simulink model "Motor_ctrl"  (R2025b)
settings: Solver=ode15s  StopTime=Tend_sim  FixedStep=Ts/10  MaxStep=Tstep  AbsTol=1e-3  EnableMultiTasking=on
InitFcn:
  | if ~exist('flagwp')
  |     tic
  |     init_sim
  | end
  | mex Motor_ctrl.c User_functions/Src/*.c
StopFcn:
  | % if ~exist('flagwp')
  |   elapsed_time=toc
  | % end
  | %plot_out_sim
values from neighbouring files (symbols this model uses):
  accel = 30000    [init_sim.m]
  Bm = 0.02    [init_sim.m]
  Clarke_inv = [1 0;-0.5 sqrt(3)/2;-0.5 -sqrt(3)/2]    [init_sim.m]
  Ctrl_strategy = 1    [init_sim.m]
  Ctrl_type = 3    [init_sim.m]
  dem = 1    [init_sim.m]
  dT = motorModel.SyreDrive.Converter.dT * 1e-6    [init_sim.m]
  EV_mode = 0    [init_sim.m]
  expC = motorModel.IronPMLossMap_dq.expC    [init_sim.m]
  expH = motorModel.IronPMLossMap_dq.expH    [init_sim.m]
  expPM = motorModel.IronPMLossMap_dq.expPM    [init_sim.m]
  Fd0 = interp2(motorModel.FluxMap_dq.Id,motorModel.FluxMap_dq.Iq,motorModel.FluxMap_dq.Fd,0,0)    [init_sim.m]
  fD_pu_norm = motorModel.FluxMapInv_dq.fD_pu_norm    [init_sim.m]
  fD_vct_max = motorModel.FluxMapInv_dq.fD_vct_max    [init_sim.m]
  fD_vct_ref = motorModel.FluxMapInv_dq.fD_vct_ref    [init_sim.m]
  Fm = interp2(Idd,Iqq,Fdd,0,0)    [init_sim.m]
  fQ_pu_norm = motorModel.FluxMapInv_dq.fQ_pu_norm    [init_sim.m]
  fQ_vct_max = motorModel.FluxMapInv_dq.fQ_vct_max    [init_sim.m]
  fQ_vct_ref = motorModel.FluxMapInv_dq.fQ_vct_ref    [init_sim.m]
  HS_ctrl = 1    [init_sim.m]
  Id_dqt = interpn(motorModel.FluxMapInv_dqt.dataF.Fd,motorModel.FluxMapInv_dqt.dataF.Fq,motorModel.FluxMapInv_dqt.dataF.th,motorModel.FluxMapInv_dqt.dataF.Id,Fd_dqt,Fq_dqt,th_dqt,'cubic')    [init_sim.m]
  Id_fe = motorModel.IronPMLossMap_dq.Id    [init_sim.m]
  iD_pu_norm = motorModel.FluxMapInv_dq.iD_pu_norm    [init_sim.m]
  idRef = interp1(abs(MTPA.id+1i*MTPA.iq),MTPA.id,i0)    [init_sim.m]
  InitIntg_d = Fm*cos(th0)    [init_sim.m]
  InitIntg_q = Fm*sin(th0)    [init_sim.m]
  inj_waveform = 1    [init_sim.m]
  Iq_dqt = interpn(motorModel.FluxMapInv_dqt.dataF.Fd,motorModel.FluxMapInv_dqt.dataF.Fq,motorModel.FluxMapInv_dqt.dataF.th,motorModel.FluxMapInv_dqt.dataF.Iq,Fd_dqt,Fq_dqt,th_dqt,'cubic')    [init_sim.m]
  Iq_fe = motorModel.IronPMLossMap_dq.Iq    [init_sim.m]
  iQ_pu_norm = motorModel.FluxMapInv_dq.iQ_pu_norm    [init_sim.m]
  iqRef = interp1(abs(MTPA.id+1i*MTPA.iq),MTPA.iq,i0)    [init_sim.m]
  IronLoss = 1    [init_sim.m]
  J = 2.7    [init_sim.m]
  motorModelType = motorModel.SyreDrive.modelSetup.motorModelType    [init_sim.m]
  n0 = motorModel.IronPMLossMap_dq.n0    [init_sim.m]
  nRef = 1000    [init_sim.m]
  p = motorModel.data.p    [init_sim.m]
  Pfe_c = motorModel.IronPMLossMap_dq.Pfes_c + motorModel.IronPMLossMap_dq.Pfer_c    [init_sim.m]
  Pfe_h = motorModel.IronPMLossMap_dq.Pfes_h + motorModel.IronPMLossMap_dq.Pfer_h    [init_sim.m]
  Ppm = motorModel.IronPMLossMap_dq.Ppm    [init_sim.m]
  Quad_Maps = 2    [init_sim.m]
  Rs = motorModel.data.Rs    [init_sim.m]
  SS_on = 1    [init_sim.m]
  T0 = interp2(motorModel.FluxMap_dq.Id,motorModel.FluxMap_dq.Iq,motorModel.FluxMap_dq.T,idRef,iqRef)    [init_sim.m]
  T_dqt = interpn(motorModel.FluxMapInv_dqt.dataF.Fd,motorModel.FluxMapInv_dqt.dataF.Fq,motorModel.FluxMapInv_dqt.dataF.th,motorModel.FluxMapInv_dqt.dataF.T,Fd_dqt,Fq_dqt,th_dqt,'cubic')    [init_sim.m]
  Tf = 6    [init_sim.m]
  th0 = 0    [init_sim.m]
  th_max = max(motorModel.FluxMapInv_dqt.dataF.th,[],'all')    [init_sim.m]
  th_min = min(motorModel.FluxMapInv_dqt.dataF.th,[],'all')    [init_sim.m]
  Ts = 1/motorModel.SyreDrive.Converter.fPWM    [init_sim.m]
  Tv = 7.1e-6    (= 7.1e-06)    [init_sim.m]
  VDC = motorModel.data.Vdc    [init_sim.m]
undefined symbols (not defined in the file or in its folder): ACloss, eMotor, interpn, J_rot, magnitude, n0_inv
libraries: nesl_utility x31, fl_lib x26, simulink x10, ee_lib x8, eeTransforms x1
(part 3 of 4)

== system Motor_ctrl/Power block - Inverter + Motor/Noncircuital/FM/Motor Model/Inverse Flux Maps/2D LUT/dq Model/SyR ==
  Vabc : Inport
  theta_elt : Inport  Port=2
  we : Inport  Port=3
  Add : Sum  Inputs=-+-
  Constant : Constant  Value=0
  Demux1 : Demux  Outputs=3
  "Fdq -> idq" : Subsystem
  Gain1 : Gain  Gain=J_rot  Multiplication=Matrix(K*u)
  Gain3 : Gain  Gain=1/p
  Integrator : Integrator  InitialCondition=[Fd0 0]
  Mux1 : Mux  Inputs=2
  Product : Product
  Product2 : Product
  Subsystem1 : Subsystem
  Terminator : Terminator
  ab->dq1 : Subsystem
      mask Display: disp('A(-theta)')
  abc->ab0 : Subsystem
  idq : Outport
  T : Outport  Port=2
  i0 : Outport  Port=3
  Fdq : Outport  Port=4
  wires:
  Subsystem1/1(SinCos) -> ab->dq1/2(sin,cos)
  Product/1 -> Add/3
  theta_elt/1 -> Gain3/1
  Mux1/1 -> ab->dq1/1(X_ab)
  Integrator/1 -> "Fdq -> idq"/1(Fdq), Fdq/1, Gain1/1
  Gain1/1 -> Product/1
  Vabc/1 -> abc->ab0/1(eabc)
  Gain3/1 -> Subsystem1/1(theta_r)
  ab->dq1/1(X_dq) -> Add/2
  abc->ab0/1(eab0) -> Demux1/1
  "Fdq -> idq"/1(idq) -> Product2/2, idq/1
  Demux1/1 -> Mux1/1
  Add/1 -> Integrator/1
  [Rs] -> Product2/1
  Demux1/2 -> Mux1/2
  "Fdq -> idq"/2(T) -> T/1
  Product2/1 -> Add/1
  we/1 -> Product/2
  Constant/1 -> i0/1
  Demux1/3 -> Terminator/1

== system Motor_ctrl/Power block - Inverter + Motor/Noncircuital/FM/Motor Model/Inverse Flux Maps/3D LUTs/Variant Subsystem/IPM ==
  Vabc : Inport
  theta_elt : Inport  Port=2
  we : Inport  Port=3
  Add : Sum  Inputs=-+-
  Constant : Constant  Value=0
  Demux1 : Demux  Outputs=3
  "Fdq -> idq" : Subsystem
      settings: PortSchema="{\"entries\":[{\"content\":{\"sides\":[{\"content\":{\"connectorIds\":[\"In1\"]},\"type\":\"ConnectorPlacement.EquallySpacedRectSide\",\"uuid\":\"c4c89702-6ed2-4f3f-ac47-63a7def21c28\"},{\"content\":{\"connectorIds\":[\"Out1\",\"Out2\"],\"side\":\"RIGHT\"},\"type\":\"ConnectorPlacement.EquallySpacedRectSide\",\"uuid\":\"78e6e96f-e01c-41b0-b9cc-2e557d2d3e77\"},{\"content\":{\"side\":\"TOP\"},\"type\":\"ConnectorPlacement.EquallySpacedRectSide\",\"uuid\":\"5ba1a012-9577-477d-841c-cd762f3f0080\"},{\"content\":{\"connectorIds\":[\"In2\"],\"side\":\"BOTTOM\"},\"type\":\"ConnectorPlacement.EquallySpacedRectSide\",\"uuid\":\"5a42fb6c-9e1a-4def-8312-83961c7d32ea\"}]},\"type\":\"ConnectorPlacement.EquallySpacedConnector\",\"uuid\":\"db03f8b0-b4f5-4aab-82fc-8dea803a4789\"}],\"packageUris\":[\"http://schema.mathworks.com/mf0/Connector/R2020b\"],\"version\":\"1.0\"}"
  Gain1 : Gain  Gain=J_rot  Multiplication=Matrix(K*u)
  Gain3 : Gain  Gain=1/p
  Integrator : Integrator  InitialCondition=[Fd0 0]
  Mux1 : Mux  Inputs=2
  Product : Product
  Product1 : Product
  Subsystem1 : Subsystem
  Terminator : Terminator
  ab->dq1 : Subsystem
      mask Display: disp('A(-theta)')
  abc->ab0 : Subsystem
  idq : Outport
  T : Outport  Port=2
  i0 : Outport  Port=3
  Fdq : Outport  Port=4
  wires:
  theta_elt/1 -> "Fdq -> idq"/2(th_e), Gain3/1
  Product1/1 -> Add/1
  Gain1/1 -> Product/1
  we/1 -> Product/2
  Product/1 -> Add/3
  Add/1 -> Integrator/1
  Integrator/1 -> Fdq/1, "Fdq -> idq"/1(Fdq), Gain1/1
  "Fdq -> idq"/1(idq) -> Product1/2, idq/1
  "Fdq -> idq"/2(T) -> T/1
  [Rs] -> Product1/1
  Vabc/1 -> abc->ab0/1(eabc)
  Gain3/1 -> Subsystem1/1(theta_r)
  abc->ab0/1(eab0) -> Demux1/1
  Subsystem1/1(SinCos) -> ab->dq1/2(sin,cos)
  Demux1/2 -> Mux1/2
  Mux1/1 -> ab->dq1/1(X_ab)
  Demux1/1 -> Mux1/1
  ab->dq1/1(X_dq) -> Add/2
  Constant/1 -> i0/1
  Demux1/3 -> Terminator/1

== system Motor_ctrl/Power block - Inverter + Motor/Noncircuital/FM/Motor Model/Inverse Flux Maps/3D LUTs/Variant Subsystem/PM-SyR ==
  Vabc : Inport
  theta_elt : Inport  Port=2
  we : Inport  Port=3
  Add : Sum  Inputs=-+-
  Constant : Constant  Value=0
  Demux1 : Demux  Outputs=3
  "Fdq -> idq" : Subsystem
      settings: PortSchema="{\"entries\":[{\"content\":{\"sides\":[{\"content\":{\"connectorIds\":[\"In1\"]},\"type\":\"ConnectorPlacement.EquallySpacedRectSide\",\"uuid\":\"658e0025-c3b4-4188-99f2-cbeabc2b5232\"},{\"content\":{\"connectorIds\":[\"Out1\",\"Out2\"],\"side\":\"RIGHT\"},\"type\":\"ConnectorPlacement.EquallySpacedRectSide\",\"uuid\":\"553a685c-efe6-4f4b-af8f-d6d55fb3aed3\"},{\"content\":{\"side\":\"TOP\"},\"type\":\"ConnectorPlacement.EquallySpacedRectSide\",\"uuid\":\"e1cc6d12-3f22-4810-870a-14518fddf4c6\"},{\"content\":{\"connectorIds\":[\"In2\"],\"side\":\"BOTTOM\"},\"type\":\"ConnectorPlacement.EquallySpacedRectSide\",\"uuid\":\"8fa353db-c23e-4667-be44-c63eaefe25e8\"}]},\"type\":\"ConnectorPlacement.EquallySpacedConnector\",\"uuid\":\"5d87f386-f61d-410e-9580-edc792fe8ce3\"}],\"packageUris\":[\"http://schema.mathworks.com/mf0/Connector/R2020b\"],\"version\":\"1.0\"}"
  Gain1 : Gain  Gain=J_rot  Multiplication=Matrix(K*u)
  Gain3 : Gain  Gain=1/p
  Integrator : Integrator  InitialCondition=[Fd0 0]
  Mux1 : Mux  Inputs=2
  Product : Product
  Product1 : Product
  Subsystem1 : Subsystem
  Terminator : Terminator
  ab->dq1 : Subsystem
      mask Display: disp('A(-theta)')
  abc->ab0 : Subsystem
  idq : Outport
  T : Outport  Port=2
  i0 : Outport  Port=3
  Fdq : Outport  Port=4
  wires:
  we/1 -> Product/2
  Subsystem1/1(SinCos) -> ab->dq1/2(sin,cos)
  Mux1/1 -> ab->dq1/1(X_ab)
  Gain1/1 -> Product/1
  Product/1 -> Add/3
  abc->ab0/1(eab0) -> Demux1/1
  ab->dq1/1(X_dq) -> Add/2
  [Rs] -> Product1/1
  "Fdq -> idq"/2(T) -> T/1
  Demux1/1 -> Mux1/1
  Product1/1 -> Add/1
  Demux1/3 -> Terminator/1
  Gain3/1 -> Subsystem1/1(theta_r)
  Integrator/1 -> "Fdq -> idq"/1(Fdq), Fdq/1, Gain1/1
  "Fdq -> idq"/1(idq) -> Product1/2, idq/1
  Demux1/2 -> Mux1/2
  Add/1 -> Integrator/1
  Vabc/1 -> abc->ab0/1(eabc)
  theta_elt/1 -> Gain3/1, "Fdq -> idq"/2(theta_elt)
  Constant/1 -> i0/1

== system Motor_ctrl/Power block - Inverter + Motor/Noncircuital/FM/Motor Model/Inverse Flux Maps/3D LUTs/Variant Subsystem/SyR ==
  Vabc : Inport
  theta_elt : Inport  Port=2
  we : Inport  Port=3
  Add : Sum  Inputs=-+-
  Constant : Constant  Value=0
  Demux1 : Demux  Outputs=3
  "Fdq -> idq" : Subsystem
      settings: PortSchema="{\"entries\":[{\"content\":{\"sides\":[{\"content\":{\"connectorIds\":[\"In1\"]},\"type\":\"ConnectorPlacement.EquallySpacedRectSide\",\"uuid\":\"658e0025-c3b4-4188-99f2-cbeabc2b5232\"},{\"content\":{\"connectorIds\":[\"Out1\",\"Out2\"],\"side\":\"RIGHT\"},\"type\":\"ConnectorPlacement.EquallySpacedRectSide\",\"uuid\":\"553a685c-efe6-4f4b-af8f-d6d55fb3aed3\"},{\"content\":{\"side\":\"TOP\"},\"type\":\"ConnectorPlacement.EquallySpacedRectSide\",\"uuid\":\"e1cc6d12-3f22-4810-870a-14518fddf4c6\"},{\"content\":{\"connectorIds\":[\"In2\"],\"side\":\"BOTTOM\"},\"type\":\"ConnectorPlacement.EquallySpacedRectSide\",\"uuid\":\"ed75ffcc-b3fe-4912-8b15-453be7565ae7\"}]},\"type\":\"ConnectorPlacement.EquallySpacedConnector\",\"uuid\":\"5d87f386-f61d-410e-9580-edc792fe8ce3\"}],\"packageUris\":[\"http://schema.mathworks.com/mf0/Connector/R2020b\"],\"version\":\"1.0\"}"
  Gain1 : Gain  Gain=J_rot  Multiplication=Matrix(K*u)
  Gain3 : Gain  Gain=1/p
  Integrator : Integrator  InitialCondition=[Fd0 0]
  Mux1 : Mux  Inputs=2
  Product : Product
  Product1 : Product
  Subsystem1 : Subsystem
  Terminator : Terminator
  ab->dq1 : Subsystem
      mask Display: disp('A(-theta)')
  abc->ab0 : Subsystem
  idq : Outport
  T : Outport  Port=2
  i0 : Outport  Port=3
  Fdq : Outport  Port=4
  wires:
  we/1 -> Product/2
  Subsystem1/1(SinCos) -> ab->dq1/2(sin,cos)
  Mux1/1 -> ab->dq1/1(X_ab)
  Gain1/1 -> Product/1
  Product/1 -> Add/3
  abc->ab0/1(eab0) -> Demux1/1
  ab->dq1/1(X_dq) -> Add/2
  [Rs] -> Product1/1
  "Fdq -> idq"/2(T) -> T/1
  Demux1/1 -> Mux1/1
  Product1/1 -> Add/1
  Gain3/1 -> Subsystem1/1(theta_r)
  Integrator/1 -> "Fdq -> idq"/1(Fdq), Fdq/1, Gain1/1
  "Fdq -> idq"/1(idq) -> Product1/2, idq/1
  Demux1/2 -> Mux1/2
  Add/1 -> Integrator/1
  Vabc/1 -> abc->ab0/1(eabc)
  theta_elt/1 -> "Fdq -> idq"/2(theta_elt), Gain3/1
  Constant/1 -> i0/1
  Demux1/3 -> Terminator/1

== system Motor_ctrl/Power block - Inverter + Motor/Noncircuital/FM/Motor Model/Iron Losses Maps/Iron Losses/Iron loss Maps/Speed Adaptation ==
  n_m : Inport
  Constant : Constant  Value=n0
  Constant1 : Constant  Value=expC
  Constant2 : Constant  Value=expH
  Constant3 : Constant  Value=expPM
  Divide : Product  Inputs=*/
  Math Function : Math  Operator=pow  SignedPower=on
  Math Function1 : Math  Operator=pow  SignedPower=on
  Math Function2 : Math  Operator=pow  SignedPower=on
  H : Outport
  C : Outport  Port=2
  PM : Outport  Port=3
  wires:
  Math Function2/1 -> PM/1
  Math Function/1 -> H/1
  Constant1/1 -> Math Function1/2
  Divide/1 -> Math Function/1, Math Function1/1, Math Function2/1
  Math Function1/1 -> C/1
  Constant/1 -> Divide/2
  Constant2/1 -> Math Function/2
  Constant3/1 -> Math Function2/2
  n_m/1 -> Divide/1

== system Motor_ctrl/Power block - Inverter + Motor/Circuital/Motor model/CCG model/Motor Model/Inverse Flux Maps/2D LUT/dq Model/IPM ==
  Fdq : Inport
  1-D Lookup Table : Lookup_n-D  NumberOfTableDimensions=1  BreakpointsForDimension1=fD_vct_ref  Table=fQ_vct_max  InternalRulePriority=Speed  RndMeth=Simplest
  Abs1 : Abs  SaturateOnIntegerOverflow=off
  Bias : Bias  Bias=-fD_vct_ref(1)  SaturateOnIntegerOverflow=off
  Constant : Constant  Value=fD_vct_ref(end)-fD_vct_ref(1)
  Demux : Demux  Outputs=2
  Divide : Product  Inputs=*/
  Divide1 : Product  Inputs=/*
  Id_pu : Lookup_n-D  BreakpointsForDimension1=fQ_pu_norm(:,1)  BreakpointsForDimension2=fD_pu_norm(1,:)  Table=iD_pu_norm  InternalRulePriority=Speed  RndMeth=Simplest
      settings: InputPortMap=u0,u1
  Iq_pu : Lookup_n-D  BreakpointsForDimension1=fQ_pu_norm(:,1)  BreakpointsForDimension2=fD_pu_norm(1,:)  Table=iQ_pu_norm  InternalRulePriority=Speed  RndMeth=Simplest
      settings: InputPortMap=u0,u1
  Mux : Mux  Inputs=2
  Product1 : Product
  Saturation : Saturate  UpperLimit=fD_vct_ref(end)  LowerLimit=fD_vct_ref(1)
  Saturation Dynamic : simulink/Discontinuities/Saturation Dynamic  OutMin=[]  OutMax=[]  OutDataTypeStr=Inherit: Same as second input  OutDataType=fixdt(1, 16)  OutScaling=2^-10  DoSatur=off
  Sign1 : Signum
  Torque calculation : Subsystem
  idq : Outport
  T : Outport  Port=2
  wires:
  Iq_pu/1 -> Product1/1
  Demux/2 -> Sign1/1, Abs1/1
  Sign1/1 -> Product1/2
  Fdq/1 -> Torque calculation/2(Fdq), Demux/1
  Mux/1 -> Torque calculation/1(Idq), idq/1
  Bias/1 -> Divide/1
  Product1/1 -> Mux/2  "iq_pu"
  Constant/1 -> Divide/2
  1-D Lookup Table/1 -> Divide1/1, Saturation Dynamic/1
  Torque calculation/1(Tm) -> T/1
  Saturation Dynamic/1 -> Divide1/2
  Abs1/1 -> Saturation Dynamic/3, Saturation Dynamic/2
  Divide1/1 -> Id_pu/1, Iq_pu/1
  Demux/1 -> Saturation/1
  Divide/1 -> Iq_pu/2, Id_pu/2
  Saturation/1 -> Bias/1, 1-D Lookup Table/1
  Id_pu/1 -> Mux/1  "iq_pu"

== system Motor_ctrl/Power block - Inverter + Motor/Circuital/Motor model/CCG model/Motor Model/Inverse Flux Maps/2D LUT/dq Model/PM-SyR ==
  Fdq : Inport
  1-D Lookup Table : Lookup_n-D  NumberOfTableDimensions=1  BreakpointsForDimension1=fQ_vct_ref  Table=fD_vct_max  InternalRulePriority=Speed  RndMeth=Simplest
  Abs : Abs  SaturateOnIntegerOverflow=off
  Bias : Bias  Bias=-fQ_vct_ref(1)  SaturateOnIntegerOverflow=off
  Constant : Constant  Value=fQ_vct_ref(end)-fQ_vct_ref(1)
  Demux : Demux  Outputs=2
  Divide : Product  Inputs=*/
  Divide1 : Product  Inputs=/*
  Id_pu : Lookup_n-D  BreakpointsForDimension1=fQ_pu_norm(:,1)  BreakpointsForDimension2=fD_pu_norm(1,:)  Table=iD_pu_norm  InternalRulePriority=Speed  RndMeth=Simplest
      settings: InputPortMap=u0,u1
  Iq_pu : Lookup_n-D  BreakpointsForDimension1=fQ_pu_norm(:,1)  BreakpointsForDimension2=fD_pu_norm(1,:)  Table=iQ_pu_norm  InternalRulePriority=Speed  RndMeth=Simplest
      settings: InputPortMap=u0,u1
  Mux : Mux  Inputs=2
  Product2 : Product
  Saturation : Saturate  UpperLimit=fQ_vct_ref(end)  LowerLimit=fQ_vct_ref(1)
  Saturation Dynamic : simulink/Discontinuities/Saturation Dynamic  OutMin=[]  OutMax=[]  OutDataTypeStr=Inherit: Same as second input  OutDataType=fixdt(1, 16)  OutScaling=2^-10  DoSatur=off
  Sign2 : Signum
  Torque calculation : Subsystem
  idq : Outport
  T : Outport  Port=2
  wires:
  Torque calculation/1(Tm) -> T/1
  Saturation/1 -> Bias/1, 1-D Lookup Table/1
  Bias/1 -> Divide/1
  Saturation Dynamic/1 -> Divide1/2
  Iq_pu/1 -> Mux/2  "iq_pu"
  1-D Lookup Table/1 -> Divide1/1, Saturation Dynamic/1
  Sign2/1 -> Product2/1
  Fdq/1 -> Torque calculation/2(Fdq), Demux/1
  Id_pu/1 -> Product2/2
  Product2/1 -> Mux/1  "id_pu"
  Mux/1 -> idq/1, Torque calculation/1(Idq)
  Constant/1 -> Divide/2
  Abs/1 -> Saturation Dynamic/3, Saturation Dynamic/2
  Demux/2 -> Saturation/1
  Demux/1 -> Sign2/1, Abs/1
  Divide1/1 -> Id_pu/2, Iq_pu/2
  Divide/1 -> Iq_pu/1, Id_pu/1

== system Motor_ctrl/Power block - Inverter + Motor/Circuital/Motor model/CCG model/Motor Model/Inverse Flux Maps/2D LUT/dq Model/SyR ==
  Fdq : Inport
  1-D Lookup Table : Lookup_n-D  NumberOfTableDimensions=1  BreakpointsForDimension1=fD_vct_ref  Table=fQ_vct_max  InternalRulePriority=Speed  RndMeth=Simplest
  Abs1 : Abs  SaturateOnIntegerOverflow=off
  Abs2 : Abs  SaturateOnIntegerOverflow=off
  Bias : Bias  Bias=-fD_vct_ref(1)  SaturateOnIntegerOverflow=off
  Constant : Constant  Value=fD_vct_ref(end)-fD_vct_ref(1)
  Demux : Demux  Outputs=2
  Divide : Product  Inputs=*/
  Divide1 : Product  Inputs=/*
  Id_pu : Lookup_n-D  BreakpointsForDimension1=fQ_pu_norm(:,1)  BreakpointsForDimension2=fD_pu_norm(1,:)  Table=iD_pu_norm  InternalRulePriority=Speed  RndMeth=Simplest
      settings: InputPortMap=u0,u1
  Iq_pu : Lookup_n-D  BreakpointsForDimension1=fQ_pu_norm(:,1)  BreakpointsForDimension2=fD_pu_norm(1,:)  Table=iQ_pu_norm  InternalRulePriority=Speed  RndMeth=Simplest
      settings: InputPortMap=u0,u1
  Mux : Mux  Inputs=2
  Product1 : Product
  Product2 : Product
  Saturation : Saturate  UpperLimit=fD_vct_ref(end)  LowerLimit=fD_vct_ref(1)
  Saturation Dynamic : simulink/Discontinuities/Saturation Dynamic  OutMin=[]  OutMax=[]  OutDataTypeStr=Inherit: Same as second input  OutDataType=fixdt(1, 16)  OutScaling=2^-10  DoSatur=off
  Sign1 : Signum
  Sign2 : Signum
  Torque calculation : Subsystem
  idq : Outport
  T : Outport  Port=2
  wires:
  Fdq/1 -> Torque calculation/2(Fdq), Demux/1
  Mux/1 -> Torque calculation/1(Idq), idq/1
  Product1/1 -> Mux/2  "iq_pu"
  Constant/1 -> Divide/2
  Bias/1 -> Divide/1
  Divide/1 -> Iq_pu/2, Id_pu/2
  Demux/2 -> Sign1/1, Abs1/1
  Saturation/1 -> Bias/1, 1-D Lookup Table/1
  Divide1/1 -> Id_pu/1, Iq_pu/1
  Demux/1 -> Abs2/1, Sign2/1
  Abs1/1 -> Saturation Dynamic/3, Saturation Dynamic/2
  Sign1/1 -> Product1/2
  Iq_pu/1 -> Product1/1
  1-D Lookup Table/1 -> Divide1/1, Saturation Dynamic/1
  Saturation Dynamic/1 -> Divide1/2
  Id_pu/1 -> Product2/2
  Product2/1 -> Mux/1  "iq_pu"
  Abs2/1 -> Saturation/1
  Sign2/1 -> Product2/1
  Torque calculation/1(Tm) -> T/1

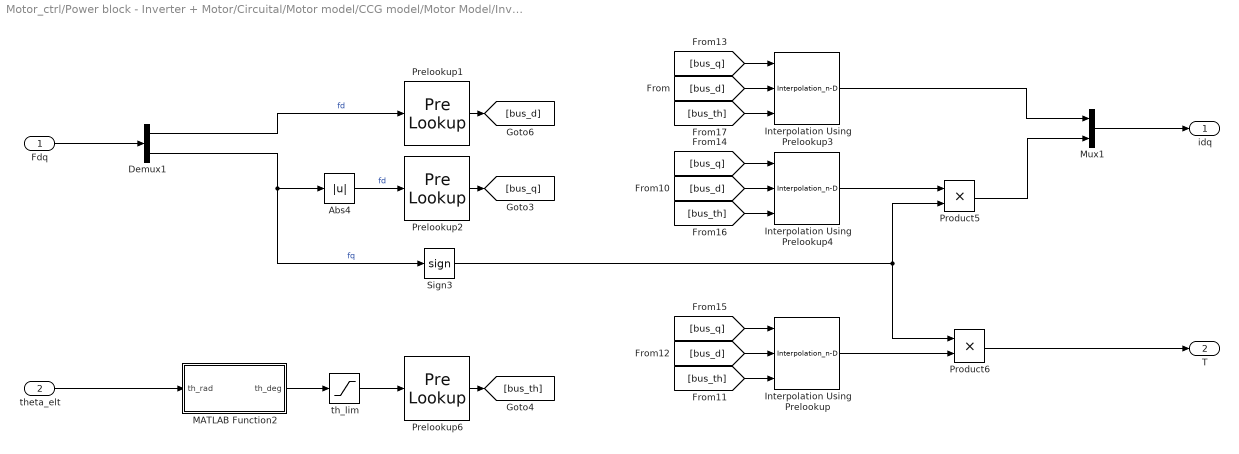
== system Motor_ctrl/Power block - Inverter + Motor/Circuital/Motor model/CCG model/Motor Model/Inverse Flux Maps/3D LUTs/Variant Subsystem/IPM ==
  Fdq : Inport
  theta_elt : Inport  Port=2
  Abs4 : Abs  SaturateOnIntegerOverflow=off
  Demux1 : Demux  Outputs=2
  Interpolation Using Prelookup : Interpolation_n-D  NumberOfTableDimensions=3  Table=T_dqt  LookupTableObject=T_th  RequireIndexFractionAsBus=on  InternalRulePriority=Speed
      settings: InputPortMap=u0,u1,u2
  Interpolation Using Prelookup3 : Interpolation_n-D  NumberOfTableDimensions=3  Table=Id_dqt  RequireIndexFractionAsBus=on  InternalRulePriority=Speed
      settings: InputPortMap=u0,u1,u2
  Interpolation Using Prelookup4 : Interpolation_n-D  NumberOfTableDimensions=3  Table=Iq_dqt  RequireIndexFractionAsBus=on  InternalRulePriority=Speed
      settings: InputPortMap=u0,u1,u2
  MATLAB Function2 : MATLAB Function  TreatAsAtomicUnit=on
  Mux1 : Mux  Inputs=2
  Prelookup1 : PreLookup  BreakpointsData=Fd_v  OutputSelection=Index and fraction as bus  ExtrapMethod=Linear
  Prelookup2 : PreLookup  BreakpointsData=Fq_v  OutputSelection=Index and fraction as bus  ExtrapMethod=Linear
  Prelookup6 : PreLookup  BreakpointsData=th_v  OutputSelection=Index and fraction as bus  ExtrapMethod=Linear
  Product5 : Product
  Product6 : Product
  Sign3 : Signum
  th_lim : Saturate  UpperLimit=th_max  LowerLimit=th_min  ZeroCross=off
  idq : Outport
  T : Outport  Port=2
  wires:
  theta_elt/1 -> MATLAB Function2/1(th_rad)
  Sign3/1 -> Product6/1, Product5/2
  Interpolation Using Prelookup3/1 -> Mux1/1
  Product5/1 -> Mux1/2
  Product6/1 -> T/1
  Interpolation Using Prelookup4/1 -> Product5/1
  Abs4/1 -> Prelookup2/1  "fd"
  MATLAB Function2/1(th_deg) -> th_lim/1
  [bus_d] -> Interpolation Using Prelookup3/2
  [bus_d] -> Interpolation Using Prelookup4/2
  Prelookup1/1 -> [bus_d]
  [bus_q] -> Interpolation Using Prelookup/1
  Demux1/2 -> Sign3/1, Abs4/1  "fq"
  [bus_th] -> Interpolation Using Prelookup/3
  [bus_q] -> Interpolation Using Prelookup4/1
  [bus_d] -> Interpolation Using Prelookup/2
  [bus_q] -> Interpolation Using Prelookup3/1
  [bus_th] -> Interpolation Using Prelookup4/3
  Demux1/1 -> Prelookup1/1  "fd"
  th_lim/1 -> Prelookup6/1
  Prelookup6/1 -> [bus_th]
  [bus_th] -> Interpolation Using Prelookup3/3
  Prelookup2/1 -> [bus_q]
  Mux1/1 -> idq/1
  Fdq/1 -> Demux1/1
  Interpolation Using Prelookup/1 -> Product6/2

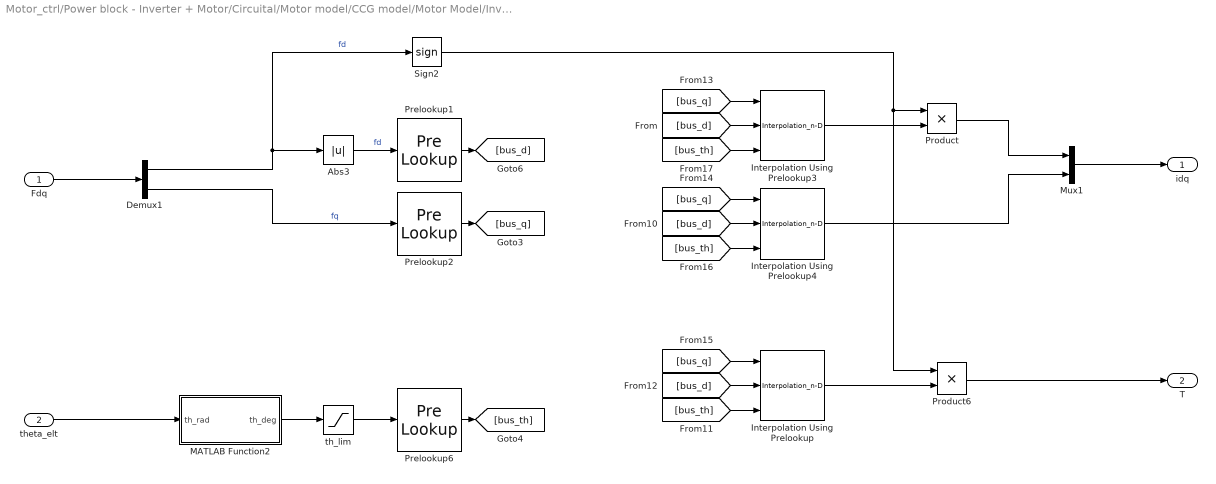
== system Motor_ctrl/Power block - Inverter + Motor/Circuital/Motor model/CCG model/Motor Model/Inverse Flux Maps/3D LUTs/Variant Subsystem/PM-SyR ==
  Fdq : Inport
  theta_elt : Inport  Port=2
  Abs3 : Abs  SaturateOnIntegerOverflow=off
  Demux1 : Demux  Outputs=2
  Interpolation Using Prelookup : Interpolation_n-D  NumberOfTableDimensions=3  Table=T_dqt  LookupTableObject=T_th  RequireIndexFractionAsBus=on  InternalRulePriority=Speed
      settings: InputPortMap=u0,u1,u2
  Interpolation Using Prelookup3 : Interpolation_n-D  NumberOfTableDimensions=3  Table=Id_dqt  RequireIndexFractionAsBus=on  InternalRulePriority=Speed
      settings: InputPortMap=u0,u1,u2
  Interpolation Using Prelookup4 : Interpolation_n-D  NumberOfTableDimensions=3  Table=Iq_dqt  RequireIndexFractionAsBus=on  InternalRulePriority=Speed
      settings: InputPortMap=u0,u1,u2
  MATLAB Function2 : MATLAB Function  TreatAsAtomicUnit=on
  Mux1 : Mux  Inputs=2
  Prelookup1 : PreLookup  BreakpointsData=Fd_v  OutputSelection=Index and fraction as bus  ExtrapMethod=Linear
  Prelookup2 : PreLookup  BreakpointsData=Fq_v  OutputSelection=Index and fraction as bus  ExtrapMethod=Linear
  Prelookup6 : PreLookup  BreakpointsData=th_v  OutputSelection=Index and fraction as bus  ExtrapMethod=Linear
  Product : Product
  Product6 : Product
  Sign2 : Signum
  th_lim : Saturate  UpperLimit=th_max  LowerLimit=th_min  ZeroCross=off
  idq : Outport
  T : Outport  Port=2
  wires:
  Sign2/1 -> Product6/1, Product/1
  Interpolation Using Prelookup3/1 -> Product/2
  ? -> ?
  theta_elt/1 -> MATLAB Function2/1(th_rad)
  Product/1 -> Mux1/1
  Interpolation Using Prelookup4/1 -> Mux1/2
  Product6/1 -> T/1
  Abs3/1 -> Prelookup1/1  "fd"
  MATLAB Function2/1(th_deg) -> th_lim/1
  [bus_d] -> Interpolation Using Prelookup3/2
  [bus_d] -> Interpolation Using Prelookup4/2
  Prelookup1/1 -> [bus_d]
  [bus_q] -> Interpolation Using Prelookup/1
  Demux1/2 -> Prelookup2/1  "fq"
  [bus_th] -> Interpolation Using Prelookup/3
  [bus_q] -> Interpolation Using Prelookup4/1
  [bus_d] -> Interpolation Using Prelookup/2
  [bus_q] -> Interpolation Using Prelookup3/1
  [bus_th] -> Interpolation Using Prelookup4/3
  Demux1/1 -> Sign2/1, Abs3/1  "fd"
  th_lim/1 -> Prelookup6/1
  Prelookup6/1 -> [bus_th]
  [bus_th] -> Interpolation Using Prelookup3/3
  Prelookup2/1 -> [bus_q]
  Mux1/1 -> idq/1
  Fdq/1 -> Demux1/1
  Interpolation Using Prelookup/1 -> Product6/2

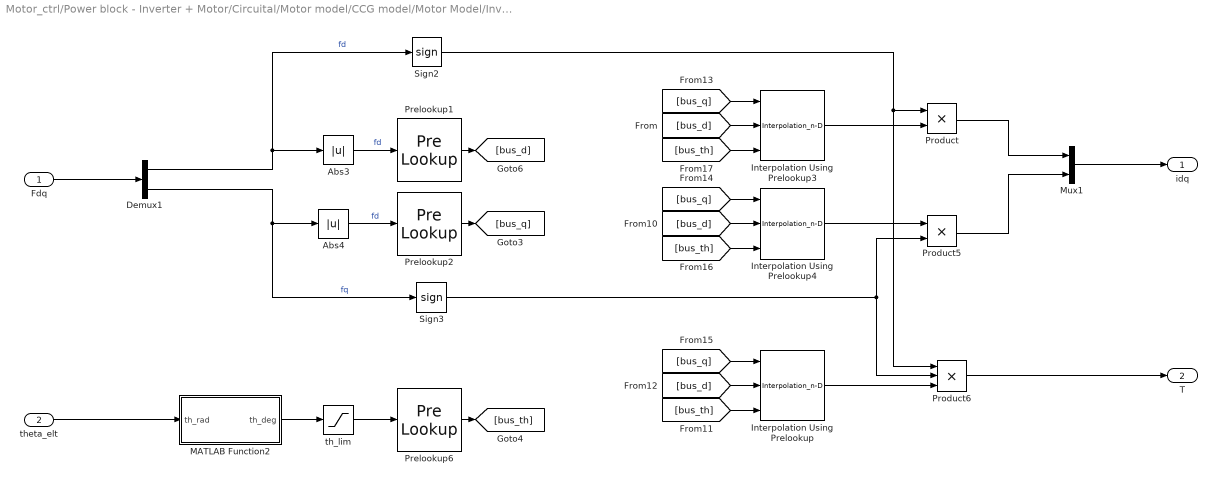
== system Motor_ctrl/Power block - Inverter + Motor/Circuital/Motor model/CCG model/Motor Model/Inverse Flux Maps/3D LUTs/Variant Subsystem/SyR ==
  Fdq : Inport
  theta_elt : Inport  Port=2
  Abs3 : Abs  SaturateOnIntegerOverflow=off
  Abs4 : Abs  SaturateOnIntegerOverflow=off
  Demux1 : Demux  Outputs=2
  Interpolation Using Prelookup : Interpolation_n-D  NumberOfTableDimensions=3  Table=T_dqt  LookupTableObject=T_th  RequireIndexFractionAsBus=on  InternalRulePriority=Speed
      settings: InputPortMap=u0,u1,u2
  Interpolation Using Prelookup3 : Interpolation_n-D  NumberOfTableDimensions=3  Table=Id_dqt  RequireIndexFractionAsBus=on  InternalRulePriority=Speed
      settings: InputPortMap=u0,u1,u2
  Interpolation Using Prelookup4 : Interpolation_n-D  NumberOfTableDimensions=3  Table=Iq_dqt  RequireIndexFractionAsBus=on  InternalRulePriority=Speed
      settings: InputPortMap=u0,u1,u2
  MATLAB Function2 : MATLAB Function  TreatAsAtomicUnit=on
  Mux1 : Mux  Inputs=2
  Prelookup1 : PreLookup  BreakpointsData=Fd_v  OutputSelection=Index and fraction as bus  ExtrapMethod=Linear
  Prelookup2 : PreLookup  BreakpointsData=Fq_v  OutputSelection=Index and fraction as bus  ExtrapMethod=Linear
  Prelookup6 : PreLookup  BreakpointsData=th_v  OutputSelection=Index and fraction as bus  ExtrapMethod=Linear
  Product : Product
  Product5 : Product
  Product6 : Product  Inputs=3
  Sign2 : Signum
  Sign3 : Signum
  th_lim : Saturate  UpperLimit=th_max  LowerLimit=th_min  ZeroCross=off
  idq : Outport
  T : Outport  Port=2
  wires:
  th_lim/1 -> Prelookup6/1
  [bus_q] -> Interpolation Using Prelookup3/1
  Demux1/1 -> Sign2/1, Abs3/1  "fd"
  Prelookup6/1 -> [bus_th]
  Prelookup2/1 -> [bus_q]
  [bus_th] -> Interpolation Using Prelookup4/3
  [bus_q] -> Interpolation Using Prelookup4/1
  Fdq/1 -> Demux1/1
  [bus_q] -> Interpolation Using Prelookup/1
  [bus_th] -> Interpolation Using Prelookup/3
  [bus_d] -> Interpolation Using Prelookup4/2
  [bus_d] -> Interpolation Using Prelookup/2
  Demux1/2 -> Sign3/1, Abs4/1  "fq"
  Prelookup1/1 -> [bus_d]
  theta_elt/1 -> MATLAB Function2/1(th_rad)
  [bus_th] -> Interpolation Using Prelookup3/3
  [bus_d] -> Interpolation Using Prelookup3/2
  MATLAB Function2/1(th_deg) -> th_lim/1
  Abs3/1 -> Prelookup1/1  "fd"
  Abs4/1 -> Prelookup2/1  "fd"
  Interpolation Using Prelookup3/1 -> Product/2
  Sign2/1 -> Product6/1, Product/1
  Interpolation Using Prelookup4/1 -> Product5/1
  Sign3/1 -> Product6/2, Product5/2
  Product/1 -> Mux1/1
  Product5/1 -> Mux1/2
  Mux1/1 -> idq/1
  Interpolation Using Prelookup/1 -> Product6/3
  Product6/1 -> T/1

== system Motor_ctrl/Power block - Inverter + Motor/Circuital/Motor model/CCG model/Motor Model/Iron Losses Maps/Iron Losses/Iron loss Maps/Speed Adaptation ==
  n_m : Inport
  Constant : Constant  Value=n0_inv
  Constant1 : Constant  Value=expC
  Constant2 : Constant  Value=expH
  Constant3 : Constant  Value=expPM
  Math Function : Math  Operator=pow  SignedPower=on
  Math Function1 : Math  Operator=pow  SignedPower=on
  Math Function2 : Math  Operator=pow  SignedPower=on
  Product : Product
  H : Outport
  C : Outport  Port=2
  PM : Outport  Port=3
  wires:
  Math Function2/1 -> PM/1
  Math Function/1 -> H/1
  Constant1/1 -> Math Function1/2
  Product/1 -> Math Function/1, Math Function1/1, Math Function2/1
  Math Function1/1 -> C/1
  Constant/1 -> Product/2
  Constant2/1 -> Math Function/2
  Constant3/1 -> Math Function2/2
  n_m/1 -> Product/1

== system Motor_ctrl/Power block - Inverter + Motor/Noncircuital/FM/Motor Model/Inverse Flux Maps/2D LUT/dq Model/IPM/Fdq -> idq ==
  Fdq : Inport
  1-D Lookup Table : Lookup_n-D  NumberOfTableDimensions=1  BreakpointsForDimension1=fD_vct_ref  Table=fQ_vct_max  InternalRulePriority=Speed  RndMeth=Simplest
  Abs1 : Abs  SaturateOnIntegerOverflow=off
  Bias : Bias  Bias=-fD_vct_ref(1)  SaturateOnIntegerOverflow=off
  Constant : Constant  Value=fD_vct_ref(end)-fD_vct_ref(1)
  Demux : Demux  Outputs=2
  Divide : Product  Inputs=*/
  Divide1 : Product  Inputs=/*
  Id_pu : Lookup_n-D  BreakpointsForDimension1=fQ_pu_norm(:,1)  BreakpointsForDimension2=fD_pu_norm(1,:)  Table=iD_pu_norm  InternalRulePriority=Speed  RndMeth=Simplest
      settings: InputPortMap=u0,u1
  Iq_pu : Lookup_n-D  BreakpointsForDimension1=fQ_pu_norm(:,1)  BreakpointsForDimension2=fD_pu_norm(1,:)  Table=iQ_pu_norm  InternalRulePriority=Speed  RndMeth=Simplest
      settings: InputPortMap=u0,u1
  Mux : Mux  Inputs=2
  Product1 : Product
  Saturation : Saturate  UpperLimit=fD_vct_ref(end)  LowerLimit=fD_vct_ref(1)
  Saturation Dynamic : simulink/Discontinuities/Saturation Dynamic  OutMin=[]  OutMax=[]  OutDataTypeStr=Inherit: Same as second input  OutDataType=fixdt(1, 16)  OutScaling=2^-10  DoSatur=off
  Sign1 : Signum
  Torque calculation : Subsystem
  idq : Outport
  T : Outport  Port=2
  wires:
  Mux/1 -> Torque calculation/1(Idq), idq/1
  Iq_pu/1 -> Product1/1
  Torque calculation/1(Tm) -> T/1
  Sign1/1 -> Product1/2
  1-D Lookup Table/1 -> Divide1/1, Saturation Dynamic/1
  Divide/1 -> Iq_pu/2, Id_pu/2
  Saturation Dynamic/1 -> Divide1/2
  Abs1/1 -> Saturation Dynamic/3, Saturation Dynamic/2
  Divide1/1 -> Id_pu/1, Iq_pu/1
  Demux/1 -> Saturation/1
  Constant/1 -> Divide/2
  Product1/1 -> Mux/2  "iq_pu"
  Demux/2 -> Sign1/1, Abs1/1
  Fdq/1 -> Torque calculation/2(Fdq), Demux/1
  Id_pu/1 -> Mux/1  "iq_pu"
  Saturation/1 -> Bias/1, 1-D Lookup Table/1
  Bias/1 -> Divide/1

== system Motor_ctrl/Power block - Inverter + Motor/Noncircuital/FM/Motor Model/Inverse Flux Maps/2D LUT/dq Model/IPM/Subsystem1 ==
  theta_r : Inport
  Gain1 : Gain  Gain=p
  Mux3 : Mux  Inputs=2
  Scope : Scope
  Scope1 : Scope
  Sin : Trigonometry
  Sin1 : Trigonometry  Operator=cos
  SinCos : Outport
  wires:
  Sin1/1 -> Mux3/2
  Sin/1 -> Mux3/1
  Mux3/1 -> Scope/1, SinCos/1
  Gain1/1 -> Scope1/1, Sin/1, Sin1/1
  theta_r/1 -> Gain1/1

== system Motor_ctrl/Power block - Inverter + Motor/Noncircuital/FM/Motor Model/Inverse Flux Maps/2D LUT/dq Model/IPM/ab->dq1 ==
  X_ab : Inport
  sin,cos : Inport  Port=2
  Demux : Demux  Outputs=2
  Demux1 : Demux  Outputs=2
  Mux : Mux  Commented=on  Inputs=2
  Mux1 : Mux  Commented=on  Inputs=2
  Mux2 : Mux  Inputs=2
  Product{,1..3} (4 alike) : Product
  Subtract : Sum
  Subtract1 : Sum  Inputs=-+
  X_d : Fcn  Commented=on  Expr=u(1)*u(4) + u(2)*u(3)
  X_q : Fcn  Commented=on  Expr=- u(1)*u(3) + u(2)*u(4)
  X_dq : Outport  InitialOutput=0
  wires:
  X_q/1 -> Mux1/2
  X_d/1 -> Mux1/1
  Mux/1 -> X_q/1, X_d/1
  Demux1/2 -> Product1/2, Product/2
  Demux/2 -> Product1/1, Product2/1
  Demux1/1 -> Product3/2, Product2/2
  Product/1 -> Subtract/1
  Product2/1 -> Subtract/2
  Demux/1 -> Product3/1, Product/1
  Product3/1 -> Subtract1/1
  Product1/1 -> Subtract1/2
  Subtract/1 -> Mux2/1
  Subtract1/1 -> Mux2/2
  X_ab/1 -> Demux/1
  sin,cos/1 -> Demux1/1
  Mux2/1 -> X_dq/1

== system Motor_ctrl/Power block - Inverter + Motor/Noncircuital/FM/Motor Model/Inverse Flux Maps/2D LUT/dq Model/IPM/abc->ab0 ==
  eabc : Inport
  Demux1 : Demux  Outputs=3
  Gain : Gain  Gain=0.5
  Gain1 : Gain  Gain=2/3
  Gain2 : Gain  Gain=1/sqrt(3)
  Gain3 : Gain  Gain=1/3
  Mux1 : Mux  Inputs=3
  Subtract : Sum  Inputs=+-
  Subtract1 : Sum
  Subtract2 : Sum  Inputs=+-
  Subtract3 : Sum  Inputs=+++
  eab0 : Outport
  wires:
  Subtract1/1 -> Gain/1
  Subtract/1 -> Gain1/1
  Demux1/2 -> Subtract3/2, Subtract2/1, Subtract1/1
  Subtract2/1 -> Gain2/1
  Subtract3/1 -> Gain3/1
  Gain1/1 -> Mux1/1
  Demux1/1 -> Subtract/1, Subtract3/1
  Gain3/1 -> Mux1/3
  Gain2/1 -> Mux1/2
  Gain/1 -> Subtract/2
  Mux1/1 -> eab0/1
  Demux1/3 -> Subtract3/3, Subtract2/2, Subtract1/2
  eabc/1 -> Demux1/1

== system Motor_ctrl/Power block - Inverter + Motor/Noncircuital/FM/Motor Model/Inverse Flux Maps/2D LUT/dq Model/PM-SyR/Fdq -> idq ==
  Fdq : Inport
  1-D Lookup Table : Lookup_n-D  NumberOfTableDimensions=1  BreakpointsForDimension1=fQ_vct_ref  Table=fD_vct_max  InternalRulePriority=Speed  RndMeth=Simplest
  Abs : Abs  SaturateOnIntegerOverflow=off
  Bias : Bias  Bias=-fQ_vct_ref(1)  SaturateOnIntegerOverflow=off
  Constant : Constant  Value=fQ_vct_ref(end)-fQ_vct_ref(1)
  Demux : Demux  Outputs=2
  Divide : Product  Inputs=*/
  Divide1 : Product  Inputs=/*
  Id_pu : Lookup_n-D  BreakpointsForDimension1=fQ_pu_norm(:,1)  BreakpointsForDimension2=fD_pu_norm(1,:)  Table=iD_pu_norm  InternalRulePriority=Speed  RndMeth=Simplest
      settings: InputPortMap=u0,u1
  Iq_pu : Lookup_n-D  BreakpointsForDimension1=fQ_pu_norm(:,1)  BreakpointsForDimension2=fD_pu_norm(1,:)  Table=iQ_pu_norm  InternalRulePriority=Speed  RndMeth=Simplest
      settings: InputPortMap=u0,u1
  Mux : Mux  Inputs=2
  Product2 : Product
  Saturation : Saturate  UpperLimit=fQ_vct_ref(end)  LowerLimit=fQ_vct_ref(1)
  Saturation Dynamic : simulink/Discontinuities/Saturation Dynamic  OutMin=[]  OutMax=[]  OutDataTypeStr=Inherit: Same as second input  OutDataType=fixdt(1, 16)  OutScaling=2^-10  DoSatur=off
  Sign2 : Signum
  Torque calculation : Subsystem
  idq : Outport
  T : Outport  Port=2
  wires:
  Sign2/1 -> Product2/1
  Constant/1 -> Divide/2
  Abs/1 -> Saturation Dynamic/3, Saturation Dynamic/2
  Iq_pu/1 -> Mux/2  "iq_pu"
  Torque calculation/1(Tm) -> T/1
  Divide/1 -> Iq_pu/1, Id_pu/1
  Bias/1 -> Divide/1
  1-D Lookup Table/1 -> Divide1/1, Saturation Dynamic/1
  Saturation/1 -> Bias/1, 1-D Lookup Table/1
  Mux/1 -> idq/1, Torque calculation/1(Idq)
  Id_pu/1 -> Product2/2
  Demux/1 -> Sign2/1, Abs/1
  Divide1/1 -> Id_pu/2, Iq_pu/2
  Demux/2 -> Saturation/1
  Fdq/1 -> Torque calculation/2(Fdq), Demux/1
  Product2/1 -> Mux/1  "id_pu"
  Saturation Dynamic/1 -> Divide1/2

== system Motor_ctrl/Power block - Inverter + Motor/Noncircuital/FM/Motor Model/Inverse Flux Maps/2D LUT/dq Model/PM-SyR/Subsystem1 ==
  theta_r : Inport
  Gain1 : Gain  Gain=p
  Mux3 : Mux  Inputs=2
  Scope : Scope
  Scope1 : Scope
  Sin : Trigonometry
  Sin1 : Trigonometry  Operator=cos
  SinCos : Outport
  wires:
  Sin1/1 -> Mux3/2
  Sin/1 -> Mux3/1
  Mux3/1 -> Scope/1, SinCos/1
  Gain1/1 -> Scope1/1, Sin/1, Sin1/1
  theta_r/1 -> Gain1/1

== system Motor_ctrl/Power block - Inverter + Motor/Noncircuital/FM/Motor Model/Inverse Flux Maps/2D LUT/dq Model/PM-SyR/ab->dq1 ==
  X_ab : Inport
  sin,cos : Inport  Port=2
  Demux : Demux  Outputs=2
  Demux1 : Demux  Outputs=2
  Mux : Mux  Commented=on  Inputs=2
  Mux1 : Mux  Commented=on  Inputs=2
  Mux2 : Mux  Inputs=2
  Product{,1..3} (4 alike) : Product
  Subtract : Sum
  Subtract1 : Sum  Inputs=-+
  X_d : Fcn  Commented=on  Expr=u(1)*u(4) + u(2)*u(3)
  X_q : Fcn  Commented=on  Expr=- u(1)*u(3) + u(2)*u(4)
  X_dq : Outport  InitialOutput=0
  wires:
  X_q/1 -> Mux1/2
  X_d/1 -> Mux1/1
  Mux/1 -> X_q/1, X_d/1
  Demux1/2 -> Product1/2, Product/2
  Demux/2 -> Product1/1, Product2/1
  Demux1/1 -> Product3/2, Product2/2
  Product/1 -> Subtract/1
  Product2/1 -> Subtract/2
  Demux/1 -> Product3/1, Product/1
  Product3/1 -> Subtract1/1
  Product1/1 -> Subtract1/2
  Subtract/1 -> Mux2/1
  Subtract1/1 -> Mux2/2
  X_ab/1 -> Demux/1
  sin,cos/1 -> Demux1/1
  Mux2/1 -> X_dq/1

== system Motor_ctrl/Power block - Inverter + Motor/Noncircuital/FM/Motor Model/Inverse Flux Maps/2D LUT/dq Model/PM-SyR/abc->ab0 ==
  eabc : Inport
  Demux1 : Demux  Outputs=3
  Gain : Gain  Gain=0.5
  Gain1 : Gain  Gain=2/3
  Gain2 : Gain  Gain=1/sqrt(3)
  Gain3 : Gain  Gain=1/3
  Mux1 : Mux  Inputs=3
  Subtract : Sum  Inputs=+-
  Subtract1 : Sum
  Subtract2 : Sum  Inputs=+-
  Subtract3 : Sum  Inputs=+++
  eab0 : Outport
  wires:
  Subtract1/1 -> Gain/1
  Subtract/1 -> Gain1/1
  Demux1/2 -> Subtract3/2, Subtract2/1, Subtract1/1
  Subtract2/1 -> Gain2/1
  Subtract3/1 -> Gain3/1
  Gain1/1 -> Mux1/1
  Demux1/1 -> Subtract/1, Subtract3/1
  Gain3/1 -> Mux1/3
  Gain2/1 -> Mux1/2
  Gain/1 -> Subtract/2
  Mux1/1 -> eab0/1
  Demux1/3 -> Subtract3/3, Subtract2/2, Subtract1/2
  eabc/1 -> Demux1/1

== system Motor_ctrl/Power block - Inverter + Motor/Noncircuital/FM/Motor Model/Inverse Flux Maps/2D LUT/dq Model/SyR/Fdq -> idq ==
  Fdq : Inport
  1-D Lookup Table : Lookup_n-D  NumberOfTableDimensions=1  BreakpointsForDimension1=fD_vct_ref  Table=fQ_vct_max  InternalRulePriority=Speed  RndMeth=Simplest
  Abs1 : Abs  SaturateOnIntegerOverflow=off
  Abs2 : Abs  SaturateOnIntegerOverflow=off
  Bias : Bias  Bias=-fD_vct_ref(1)  SaturateOnIntegerOverflow=off
  Constant : Constant  Value=fD_vct_ref(end)-fD_vct_ref(1)
  Demux : Demux  Outputs=2
  Divide : Product  Inputs=*/
  Divide1 : Product  Inputs=/*
  Id_pu : Lookup_n-D  BreakpointsForDimension1=fQ_pu_norm(:,1)  BreakpointsForDimension2=fD_pu_norm(1,:)  Table=iD_pu_norm  InternalRulePriority=Speed  RndMeth=Simplest
      settings: InputPortMap=u0,u1
  Iq_pu : Lookup_n-D  BreakpointsForDimension1=fQ_pu_norm(:,1)  BreakpointsForDimension2=fD_pu_norm(1,:)  Table=iQ_pu_norm  InternalRulePriority=Speed  RndMeth=Simplest
      settings: InputPortMap=u0,u1
  Mux : Mux  Inputs=2
  Product1 : Product
  Product2 : Product
  Saturation : Saturate  UpperLimit=fD_vct_ref(end)  LowerLimit=fD_vct_ref(1)
  Saturation Dynamic : simulink/Discontinuities/Saturation Dynamic  OutMin=[]  OutMax=[]  OutDataTypeStr=Inherit: Same as second input  OutDataType=fixdt(1, 16)  OutScaling=2^-10  DoSatur=off
  Sign1 : Signum
  Sign2 : Signum
  Torque calculation : Subsystem
  idq : Outport
  T : Outport  Port=2
  wires:
  1-D Lookup Table/1 -> Divide1/1, Saturation Dynamic/1
  Divide/1 -> Iq_pu/2, Id_pu/2
  Torque calculation/1(Tm) -> T/1
  Abs1/1 -> Saturation Dynamic/3, Saturation Dynamic/2
  Fdq/1 -> Torque calculation/2(Fdq), Demux/1
  Demux/2 -> Sign1/1, Abs1/1
  Iq_pu/1 -> Product1/1
  Abs2/1 -> Saturation/1
  Saturation/1 -> Bias/1, 1-D Lookup Table/1
  Divide1/1 -> Id_pu/1, Iq_pu/1
  Id_pu/1 -> Product2/2
  Bias/1 -> Divide/1
  Saturation Dynamic/1 -> Divide1/2
  Constant/1 -> Divide/2
  Sign1/1 -> Product1/2
  Mux/1 -> Torque calculation/1(Idq), idq/1
  Demux/1 -> Abs2/1, Sign2/1
  Product2/1 -> Mux/1  "iq_pu"
  Sign2/1 -> Product2/1
  Product1/1 -> Mux/2  "iq_pu"

== system Motor_ctrl/Power block - Inverter + Motor/Noncircuital/FM/Motor Model/Inverse Flux Maps/2D LUT/dq Model/SyR/Subsystem1 ==
  theta_r : Inport
  Gain1 : Gain  Gain=p
  Mux3 : Mux  Inputs=2
  Scope : Scope
  Scope1 : Scope
  Sin : Trigonometry
  Sin1 : Trigonometry  Operator=cos
  SinCos : Outport
  wires:
  Sin1/1 -> Mux3/2
  Sin/1 -> Mux3/1
  Mux3/1 -> Scope/1, SinCos/1
  Gain1/1 -> Scope1/1, Sin/1, Sin1/1
  theta_r/1 -> Gain1/1

== system Motor_ctrl/Power block - Inverter + Motor/Noncircuital/FM/Motor Model/Inverse Flux Maps/2D LUT/dq Model/SyR/ab->dq1 ==
  X_ab : Inport
  sin,cos : Inport  Port=2
  Demux : Demux  Outputs=2
  Demux1 : Demux  Outputs=2
  Mux : Mux  Commented=on  Inputs=2
  Mux1 : Mux  Commented=on  Inputs=2
  Mux2 : Mux  Inputs=2
  Product{,1..3} (4 alike) : Product
  Subtract : Sum
  Subtract1 : Sum  Inputs=-+
  X_d : Fcn  Commented=on  Expr=u(1)*u(4) + u(2)*u(3)
  X_q : Fcn  Commented=on  Expr=- u(1)*u(3) + u(2)*u(4)
  X_dq : Outport  InitialOutput=0
  wires:
  X_q/1 -> Mux1/2
  X_d/1 -> Mux1/1
  Mux/1 -> X_q/1, X_d/1
  Demux1/2 -> Product1/2, Product/2
  Demux/2 -> Product1/1, Product2/1
  Demux1/1 -> Product3/2, Product2/2
  Product/1 -> Subtract/1
  Product2/1 -> Subtract/2
  Demux/1 -> Product3/1, Product/1
  Product3/1 -> Subtract1/1
  Product1/1 -> Subtract1/2
  Subtract/1 -> Mux2/1
  Subtract1/1 -> Mux2/2
  X_ab/1 -> Demux/1
  sin,cos/1 -> Demux1/1
  Mux2/1 -> X_dq/1

== system Motor_ctrl/Power block - Inverter + Motor/Noncircuital/FM/Motor Model/Inverse Flux Maps/2D LUT/dq Model/SyR/abc->ab0 ==
  eabc : Inport
  Demux1 : Demux  Outputs=3
  Gain : Gain  Gain=0.5
  Gain1 : Gain  Gain=2/3
  Gain2 : Gain  Gain=1/sqrt(3)
  Gain3 : Gain  Gain=1/3
  Mux1 : Mux  Inputs=3
  Subtract : Sum  Inputs=+-
  Subtract1 : Sum
  Subtract2 : Sum  Inputs=+-
  Subtract3 : Sum  Inputs=+++
  eab0 : Outport
  wires:
  Subtract1/1 -> Gain/1
  Subtract/1 -> Gain1/1
  Demux1/2 -> Subtract3/2, Subtract2/1, Subtract1/1
  Subtract2/1 -> Gain2/1
  Subtract3/1 -> Gain3/1
  Gain1/1 -> Mux1/1
  Demux1/1 -> Subtract/1, Subtract3/1
  Gain3/1 -> Mux1/3
  Gain2/1 -> Mux1/2
  Gain/1 -> Subtract/2
  Mux1/1 -> eab0/1
  Demux1/3 -> Subtract3/3, Subtract2/2, Subtract1/2
  eabc/1 -> Demux1/1

== system Motor_ctrl/Power block - Inverter + Motor/Noncircuital/FM/Motor Model/Inverse Flux Maps/3D LUTs/Variant Subsystem/IPM/Fdq -> idq ==
  Fdq : Inport
  th_e : Inport  Port=2
  Abs4 : Abs  SaturateOnIntegerOverflow=off
  Demux1 : Demux  Outputs=2
  Interpolation Using Prelookup : Interpolation_n-D  NumberOfTableDimensions=3  Table=T_dqt  LookupTableObject=T_th  RequireIndexFractionAsBus=on  InternalRulePriority=Speed
      settings: InputPortMap=u0,u1,u2
  Interpolation Using Prelookup3 : Interpolation_n-D  NumberOfTableDimensions=3  Table=Id_dqt  RequireIndexFractionAsBus=on  InternalRulePriority=Speed
      settings: InputPortMap=u0,u1,u2
  Interpolation Using Prelookup4 : Interpolation_n-D  NumberOfTableDimensions=3  Table=Iq_dqt  RequireIndexFractionAsBus=on  InternalRulePriority=Speed
      settings: InputPortMap=u0,u1,u2
  MATLAB Function2 : MATLAB Function  TreatAsAtomicUnit=on
  Mux1 : Mux  Inputs=2
  Prelookup1 : PreLookup  BreakpointsData=Fd_v  OutputSelection=Index and fraction as bus  BeginIndexSearchUsingPreviousIndexResult=on  ExtrapMethod=Linear
  Prelookup2 : PreLookup  BreakpointsData=Fq_v  OutputSelection=Index and fraction as bus  BeginIndexSearchUsingPreviousIndexResult=on  ExtrapMethod=Linear
  Prelookup6 : PreLookup  BreakpointsData=th_v  OutputSelection=Index and fraction as bus  ExtrapMethod=Linear
  Product1 : Product
  Product5 : Product
  Sign3 : Signum
  th_lim : Saturate  UpperLimit=th_max  LowerLimit=th_min  ZeroCross=off
  idq : Outport
  T : Outport  Port=2
  wires:
  [bus_q] -> Interpolation Using Prelookup4/1
  Product5/1 -> Mux1/2
  Demux1/1 -> Prelookup1/1  "fd"
  [bus_d] -> Interpolation Using Prelookup3/2
  Demux1/2 -> Sign3/1, Abs4/1  "fq"
  Sign3/1 -> Product5/2, Product1/1
  Interpolation Using Prelookup4/1 -> Product5/1
  Interpolation Using Prelookup3/1 -> Mux1/1
  Prelookup2/1 -> [bus_q]
  Abs4/1 -> Prelookup2/1  "fd"
  Mux1/1 -> idq/1
  Prelookup1/1 -> [bus_d]
  [bus_d] -> Interpolation Using Prelookup4/2
  [bus_q] -> Interpolation Using Prelookup3/1
  Fdq/1 -> Demux1/1
  [bus_q] -> Interpolation Using Prelookup/1
  [bus_d] -> Interpolation Using Prelookup/2
  Interpolation Using Prelookup/1 -> Product1/2
  Product1/1 -> T/1
  th_lim/1 -> Prelookup6/1
  MATLAB Function2/1(th_deg) -> th_lim/1
  th_e/1 -> MATLAB Function2/1(th_rad)
  Prelookup6/1 -> [bus_th]
  [bus_th] -> Interpolation Using Prelookup/3
  [bus_th] -> Interpolation Using Prelookup4/3
  [bus_th] -> Interpolation Using Prelookup3/3

== system Motor_ctrl/Power block - Inverter + Motor/Noncircuital/FM/Motor Model/Inverse Flux Maps/3D LUTs/Variant Subsystem/IPM/Subsystem1 ==
  theta_r : Inport
  Gain1 : Gain  Gain=p
  Mux3 : Mux  Inputs=2
  Scope : Scope
  Scope1 : Scope
  Sin : Trigonometry
  Sin1 : Trigonometry  Operator=cos
  SinCos : Outport
  wires:
  Sin1/1 -> Mux3/2
  Sin/1 -> Mux3/1
  Mux3/1 -> Scope/1, SinCos/1
  Gain1/1 -> Scope1/1, Sin/1, Sin1/1
  theta_r/1 -> Gain1/1

== system Motor_ctrl/Power block - Inverter + Motor/Noncircuital/FM/Motor Model/Inverse Flux Maps/3D LUTs/Variant Subsystem/IPM/ab->dq1 ==
  X_ab : Inport
  sin,cos : Inport  Port=2
  Demux : Demux  Outputs=2
  Demux1 : Demux  Outputs=2
  Mux : Mux  Commented=on  Inputs=2
  Mux1 : Mux  Commented=on  Inputs=2
  Mux2 : Mux  Inputs=2
  Product{,1..3} (4 alike) : Product
  Subtract : Sum
  Subtract1 : Sum  Inputs=-+
  X_d : Fcn  Commented=on  Expr=u(1)*u(4) + u(2)*u(3)
  X_q : Fcn  Commented=on  Expr=- u(1)*u(3) + u(2)*u(4)
  X_dq : Outport  InitialOutput=0
  wires:
  X_q/1 -> Mux1/2
  X_d/1 -> Mux1/1
  Mux/1 -> X_q/1, X_d/1
  Demux1/2 -> Product1/2, Product/2
  Demux/2 -> Product1/1, Product2/1
  Demux1/1 -> Product3/2, Product2/2
  Product/1 -> Subtract/1
  Product2/1 -> Subtract/2
  Demux/1 -> Product3/1, Product/1
  Product3/1 -> Subtract1/1
  Product1/1 -> Subtract1/2
  Subtract/1 -> Mux2/1
  Subtract1/1 -> Mux2/2
  X_ab/1 -> Demux/1
  sin,cos/1 -> Demux1/1
  Mux2/1 -> X_dq/1

== system Motor_ctrl/Power block - Inverter + Motor/Noncircuital/FM/Motor Model/Inverse Flux Maps/3D LUTs/Variant Subsystem/IPM/abc->ab0 ==
  eabc : Inport
  Demux1 : Demux  Outputs=3
  Gain : Gain  Gain=0.5
  Gain1 : Gain  Gain=2/3
  Gain2 : Gain  Gain=1/sqrt(3)
  Gain3 : Gain  Gain=1/3
  Mux1 : Mux  Inputs=3
  Subtract : Sum  Inputs=+-
  Subtract1 : Sum
  Subtract2 : Sum  Inputs=+-
  Subtract3 : Sum  Inputs=+++
  eab0 : Outport
  wires:
  Subtract1/1 -> Gain/1
  Subtract/1 -> Gain1/1
  Demux1/2 -> Subtract3/2, Subtract2/1, Subtract1/1
  Subtract2/1 -> Gain2/1
  Subtract3/1 -> Gain3/1
  Gain1/1 -> Mux1/1
  Demux1/1 -> Subtract/1, Subtract3/1
  Gain3/1 -> Mux1/3
  Gain2/1 -> Mux1/2
  Gain/1 -> Subtract/2
  Mux1/1 -> eab0/1
  Demux1/3 -> Subtract3/3, Subtract2/2, Subtract1/2
  eabc/1 -> Demux1/1

== system Motor_ctrl/Power block - Inverter + Motor/Noncircuital/FM/Motor Model/Inverse Flux Maps/3D LUTs/Variant Subsystem/PM-SyR/Fdq -> idq ==
  Fdq : Inport
  theta_elt : Inport  Port=2
  Abs3 : Abs  SaturateOnIntegerOverflow=off
  Demux1 : Demux  Outputs=2
  Interpolation Using Prelookup : Interpolation_n-D  NumberOfTableDimensions=3  Table=T_dqt  LookupTableObject=T_th  RequireIndexFractionAsBus=on  InternalRulePriority=Speed
      settings: InputPortMap=u0,u1,u2
  Interpolation Using Prelookup3 : Interpolation_n-D  NumberOfTableDimensions=3  Table=Id_dqt  RequireIndexFractionAsBus=on  InternalRulePriority=Speed
      settings: InputPortMap=u0,u1,u2
  Interpolation Using Prelookup4 : Interpolation_n-D  NumberOfTableDimensions=3  Table=Iq_dqt  RequireIndexFractionAsBus=on  InternalRulePriority=Speed
      settings: InputPortMap=u0,u1,u2
  MATLAB Function2 : MATLAB Function  TreatAsAtomicUnit=on
  Mux1 : Mux  Inputs=2
  Prelookup1 : PreLookup  BreakpointsData=Fd_v  OutputSelection=Index and fraction as bus  ExtrapMethod=Linear
  Prelookup2 : PreLookup  BreakpointsData=Fq_v  OutputSelection=Index and fraction as bus  ExtrapMethod=Linear
  Prelookup6 : PreLookup  BreakpointsData=th_v  OutputSelection=Index and fraction as bus  ExtrapMethod=Linear
  Product : Product
  Product6 : Product
  Sign2 : Signum
  th_lim : Saturate  UpperLimit=th_max  LowerLimit=th_min  ZeroCross=off
  idq : Outport
  T : Outport  Port=2
  wires:
  Sign2/1 -> Product6/1, Product/1
  [bus_d] -> Interpolation Using Prelookup/2
  [bus_th] -> Interpolation Using Prelookup/3
  Interpolation Using Prelookup4/1 -> Mux1/2
  theta_elt/1 -> MATLAB Function2/1(th_rad)
  Mux1/1 -> idq/1
  Fdq/1 -> Demux1/1
  Prelookup6/1 -> [bus_th]
  Prelookup2/1 -> [bus_q]
  Abs3/1 -> Prelookup1/1  "fd"
  Product6/1 -> T/1
  [bus_d] -> Interpolation Using Prelookup3/2
  [bus_th] -> Interpolation Using Prelookup4/3
  [bus_q] -> Interpolation Using Prelookup/1
  [bus_q] -> Interpolation Using Prelookup4/1
  Interpolation Using Prelookup3/1 -> Product/2
  MATLAB Function2/1(th_deg) -> th_lim/1
  Product/1 -> Mux1/1
  [bus_th] -> Interpolation Using Prelookup3/3
  Demux1/2 -> Prelookup2/1  "fq"
  [bus_q] -> Interpolation Using Prelookup3/1
  [bus_d] -> Interpolation Using Prelookup4/2
  th_lim/1 -> Prelookup6/1
  Interpolation Using Prelookup/1 -> Product6/2
  Demux1/1 -> Sign2/1, Abs3/1  "fd"
  Prelookup1/1 -> [bus_d]
  ? -> ?

== system Motor_ctrl/Power block - Inverter + Motor/Noncircuital/FM/Motor Model/Inverse Flux Maps/3D LUTs/Variant Subsystem/PM-SyR/Subsystem1 ==
  theta_r : Inport
  Gain1 : Gain  Gain=p
  Mux3 : Mux  Inputs=2
  Scope : Scope
  Scope1 : Scope
  Sin : Trigonometry
  Sin1 : Trigonometry  Operator=cos
  SinCos : Outport
  wires:
  Sin1/1 -> Mux3/2
  Sin/1 -> Mux3/1
  Mux3/1 -> Scope/1, SinCos/1
  Gain1/1 -> Scope1/1, Sin/1, Sin1/1
  theta_r/1 -> Gain1/1

== system Motor_ctrl/Power block - Inverter + Motor/Noncircuital/FM/Motor Model/Inverse Flux Maps/3D LUTs/Variant Subsystem/PM-SyR/ab->dq1 ==
  X_ab : Inport
  sin,cos : Inport  Port=2
  Demux : Demux  Outputs=2
  Demux1 : Demux  Outputs=2
  Mux : Mux  Commented=on  Inputs=2
  Mux1 : Mux  Commented=on  Inputs=2
  Mux2 : Mux  Inputs=2
  Product{,1..3} (4 alike) : Product
  Subtract : Sum
  Subtract1 : Sum  Inputs=-+
  X_d : Fcn  Commented=on  Expr=u(1)*u(4) + u(2)*u(3)
  X_q : Fcn  Commented=on  Expr=- u(1)*u(3) + u(2)*u(4)
  X_dq : Outport  InitialOutput=0
  wires:
  X_q/1 -> Mux1/2
  X_d/1 -> Mux1/1
  Mux/1 -> X_q/1, X_d/1
  Demux1/2 -> Product1/2, Product/2
  Demux/2 -> Product1/1, Product2/1
  Demux1/1 -> Product3/2, Product2/2
  Product/1 -> Subtract/1
  Product2/1 -> Subtract/2
  Demux/1 -> Product3/1, Product/1
  Product3/1 -> Subtract1/1
  Product1/1 -> Subtract1/2
  Subtract/1 -> Mux2/1
  Subtract1/1 -> Mux2/2
  X_ab/1 -> Demux/1
  sin,cos/1 -> Demux1/1
  Mux2/1 -> X_dq/1

== system Motor_ctrl/Power block - Inverter + Motor/Noncircuital/FM/Motor Model/Inverse Flux Maps/3D LUTs/Variant Subsystem/PM-SyR/abc->ab0 ==
  eabc : Inport
  Demux1 : Demux  Outputs=3
  Gain : Gain  Gain=0.5
  Gain1 : Gain  Gain=2/3
  Gain2 : Gain  Gain=1/sqrt(3)
  Gain3 : Gain  Gain=1/3
  Mux1 : Mux  Inputs=3
  Subtract : Sum  Inputs=+-
  Subtract1 : Sum
  Subtract2 : Sum  Inputs=+-
  Subtract3 : Sum  Inputs=+++
  eab0 : Outport
  wires:
  Subtract1/1 -> Gain/1
  Subtract/1 -> Gain1/1
  Demux1/2 -> Subtract3/2, Subtract2/1, Subtract1/1
  Subtract2/1 -> Gain2/1
  Subtract3/1 -> Gain3/1
  Gain1/1 -> Mux1/1
  Demux1/1 -> Subtract/1, Subtract3/1
  Gain3/1 -> Mux1/3
  Gain2/1 -> Mux1/2
  Gain/1 -> Subtract/2
  Mux1/1 -> eab0/1
  Demux1/3 -> Subtract3/3, Subtract2/2, Subtract1/2
  eabc/1 -> Demux1/1
